simulink model "hydraulic_system_sim"  (R2021b)
settings: Solver=VariableStepAuto  StartTime=0.0  StopTime=10.0  RelTol=1e-3
values from neighbouring files (symbols this model uses):
  del_p = 70    [hydraulic_system.m]
  e_h = (rho_g/A) * (1e-6/132)    (= 0.964575412678)    [hydraulic_system.m]
  l_p = 20e-3    (= 0.02)    [hydraulic_system.m]
  r_s = (del_p/5)*60e-3    (= 0.84)    [hydraulic_system.m]
  w_n_sq = 2*e_h/l_p    (= 96.4575412678)    [hydraulic_system.m]
libraries: slpidlib x1
settings Model: Creator=eraym  LastModifiedBy=eraym

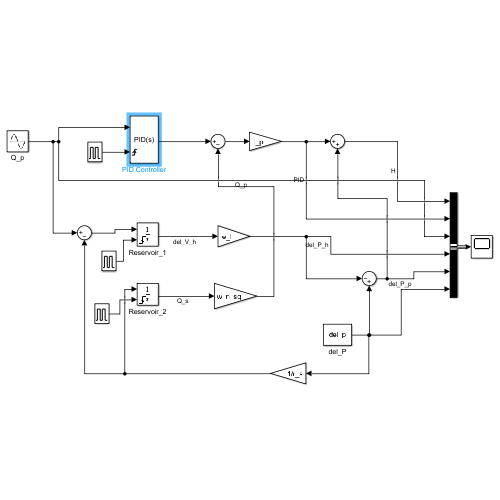
[thumbnail: Simulink's stored preview of the top-level diagram]
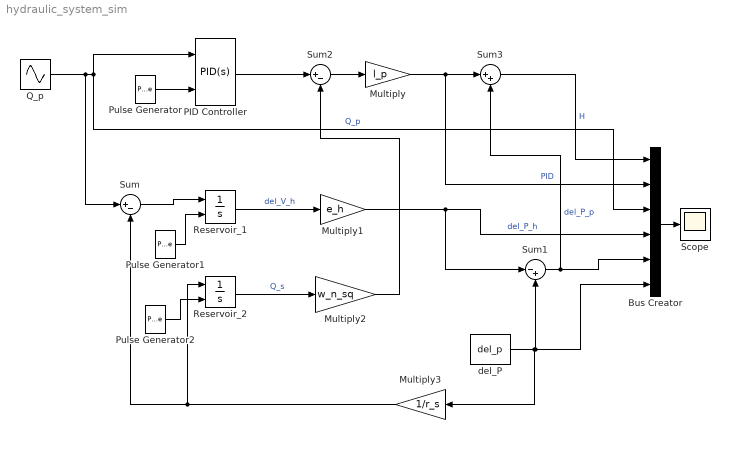
== system hydraulic_system_sim ==
  Bus Creator : BusCreator  Inputs=6
  Multiply : Gain  Gain=l_p
  Multiply1 : Gain  Gain=e_h
  Multiply2 : Gain  Gain=w_n_sq
  Multiply3 : Gain  Gain=1/r_s
  PID Controller : slpidlib/PID Controller  Controller=PID  Form=Parallel  TimeDomain=Continuous-time  UseExternalTs=off  SampleTime=-1  IntegratorMethod=Forward Euler  FilterMethod=Forward Euler  ControllerParametersSource=internal  P=-10050  I=-2  D=100  UseFilter=on  N=100  TunerSelectOption=Frequency Response Based  InitialConditionSource=internal  InitialConditionForIntegrator=0  InitialConditionForFilter=0  DifferentiatorICPrevScaledInput=0  ExternalReset=rising  TrackingMode=off  Kt=1  LimitOutput=off  SatLimitsSource=internal  UpperSaturationLimit=inf  LowerSaturationLimit=-inf  LinearizeAsGain=on  AntiWindupMode=none  Kb=1  POutMin=[]  POutMax=[]  IOutMin=[]  IOutMax=[]  DOutMin=[]  DOutMax=[]  NOutMin=[]  NOutMax=[]  SumOutMin=[]  SumOutMax=[]  SaturationOutMin=[]  SaturationOutMax=[]  PParamMin=[]  PParamMax=[]  IParamMin=[]  IParamMax=[]  DParamMin=[]  DParamMax=[]  NParamMin=[]  NParamMax=[]  KbParamMin=[]  KbParamMax=[]  KtParamMin=[]  KtParamMax=[]  KbOutMin=[]  KbOutMax=[]  KtOutMin=[]  KtOutMax=[]  IntegratorOutMin=[]  IntegratorOutMax=[]  FilterOutMin=[]  FilterOutMax=[]  SumI1OutMin=[]  SumI1OutMax=[]  SumI2OutMin=[]  SumI2OutMax=[]  SumI3OutMin=[]  SumI3OutMax=[]  SumI4OutMin=[]  SumI4OutMax=[]  SumDOutMin=[]  SumDOutMax=[]  DifferentiatorOutMin=[]  DifferentiatorOutMax=[]  FilterDiffOutCoefMin=[]  FilterDiffOutCoefMax=[]  ReciprocalOutMin=[]  ReciprocalOutMax=[]  SumDenOutMin=[]  SumDenOutMax=[]  SumNumOutMin=[]  SumNumOutMax=[]  DivideOutMin=[]  DivideOutMax=[]  UdiffTsProdOutMin=[]  UdiffTsProdOutMax=[]  NTsProdOutMin=[]  NTsProdOutMax=[]  UintegralTsProdOutMin=[]  UintegralTsProdOutMax=[]  UngainTsProdOutMin=[]  UngainTsProdOutMax=[]  IntegratorContinuousStateAttributes=''  IntegratorStateMustResolveToSignalObject=off  IntegratorRTWStateStorageClass=Auto  FilterContinuousStateAttributes=''  FilterStateMustResolveToSignalObject=off  FilterRTWStateStorageClass=Auto  ParallelPVariant=InternalParameters  IdealPVariant=Disabled  IVariant=InternalParameters  DVariant=InternalParameters  IntegratorVariant=Continuous  SatVariant=Disabled  AWVariant=Passthrough  PCopyVariant=Disabled  TRVariant=Disabled  FdbkBlocksVariant=Forward  IdealPFdbkVariant=Disabled  SatFdbkVariant=Disabled  DerivativeFilterVariant=ContFilter  NVariant=InternalParameters  NCopyVariant=Disabled  FilterICVariant=InternalICsFilter  IntegratorICVariant=InternalICs  ExternalResetVariant=ExternalReset  TRSumVariant=Passthrough  SumFdbkVariant=Disabled  SumVariant=Sum_PID  TsampFilterVariant=InternalTs  TsampNgainVariant=Passthrough  TsampIntegralVariant=Passthrough  ExternalSaturationOutDataTypeStr=Inherit: Same as second input
  Pulse Generator : DiscretePulseGenerator  PulseType=Time based  Period=1
  Pulse Generator1 : DiscretePulseGenerator  PulseType=Time based  Period=1
  Pulse Generator2 : DiscretePulseGenerator  PulseType=Time based  Period=1
  Q_p : Sin  Amplitude=10  Bias=90  Frequency=6.5  SampleTime=0
  Reservoir_1 : Integrator  ExternalReset=rising
  Reservoir_2 : Integrator  ExternalReset=rising
  Scope : Scope
  Sum : Sum  Inputs=|+-
  Sum1 : Sum  Inputs=|-+
  Sum2 : Sum  Inputs=|+-
  Sum3 : Sum  Inputs=|++
  del_P : Constant  Value=del_p
  wires:
  Q_p/1 -> PID Controller/1, Bus Creator/3, Sum/1  "Q_p"
  Reservoir_1/1 -> Multiply1/1  "del_V_h"
  Reservoir_2/1 -> Multiply2/1  "Q_s"
  Sum/1 -> Reservoir_1/1
  del_P/1 -> Bus Creator/6, Sum1/2, Multiply3/1
  Sum1/1 -> Bus Creator/5, Sum3/2  "del_P_p"
  Multiply1/1 -> Bus Creator/4, Sum1/1  "del_P_h"
  Multiply2/1 -> Sum2/2
  Sum2/1 -> Multiply/1
  Multiply/1 -> Bus Creator/2, Sum3/1  "PID"
  Sum3/1 -> Bus Creator/1  "H"
  Multiply3/1 -> Reservoir_2/1, Sum/2
  Pulse Generator1/1 -> Reservoir_1/2
  Pulse Generator2/1 -> Reservoir_2/2
  Bus Creator/1 -> Scope/1
  PID Controller/1 -> Sum2/1
  Pulse Generator/1 -> PID Controller/2
